simulink model "EPA_Jumpe_v1"  (R2018a)
settings: Solver=FixedStepDiscrete  StartTime=0.0  StopTime=inf  FixedStep=0.001  RelTol=1e-3  EnableMultiTasking=on
model workspace (MAT data in the model file):
  MCOS : class17 (value not decoded)
values from neighbouring files (symbols this model uses):
  bits_current = 12    [Init_EPA_Jumper.m]
  bits_GRF = 12    [Init_EPA_Jumper.m]
  bits_Kd = 12    [Init_EPA_Jumper.m]
  bits_Kp = 12    [Init_EPA_Jumper.m]
  bits_position = 16    [Init_EPA_Jumper.m]
  bits_velocity = 12    [Init_EPA_Jumper.m]
  deadzone_in_TIB = 0.45    [Init_EPA_Jumper.m]
  deadzone_out_TIB = 0.48    [Init_EPA_Jumper.m]
  GRF_MAX = 3.3    [Init_EPA_Jumper.m]
  GRF_MIN = 0    [Init_EPA_Jumper.m]
  k_p_TIB = 1    [Init_EPA_Jumper.m]
  KD_MAX = 5.0    (= 5)    [Init_EPA_Jumper.m]
  KD_MIN = 0.0    (= 0)    [Init_EPA_Jumper.m]
  KP_MAX = 500.0    (= 500)    [Init_EPA_Jumper.m]
  KP_MIN = 0.0    (= 0)    [Init_EPA_Jumper.m]
  P_MAX = 95.5    [Init_EPA_Jumper.m]
  P_MIN = -95.5    [Init_EPA_Jumper.m]
  PressureFilter_CutOffFreq = 50    [Init_EPA_Jumper.m]
  PressureFilter_Gain = 1    [Init_EPA_Jumper.m]
  ReadingVoltage = 5    [Init_EPA_Jumper.m]
  T_MAX = 18.0    (= 18)    [Init_EPA_Jumper.m]
  T_MIN = -18.0    (= -18)    [Init_EPA_Jumper.m]
  V_MAX = 45.0    (= 45)    [Init_EPA_Jumper.m]
  V_MIN = -45.0    (= -45)    [Init_EPA_Jumper.m]
  voltageBias_GAS = -2.3721    [Init_EPA_Jumper.m]
  voltageBias_GL = -2.2892    [Init_EPA_Jumper.m]
  voltageBias_HAM = -2.3721    [Init_EPA_Jumper.m]
  voltageBias_IL = -2.3721    [Init_EPA_Jumper.m]
  voltageBias_POP = -2.3721    [Init_EPA_Jumper.m]
  voltageBias_RF = -2.3721    [Init_EPA_Jumper.m]
  voltageBias_SOL = -2.3721    [Init_EPA_Jumper.m]
  voltageBias_TIB = -2.3721    [Init_EPA_Jumper.m]
  voltageBias_VAS = -2.3721    [Init_EPA_Jumper.m]
  voltageMultiplier_GAS = 2.4915    [Init_EPA_Jumper.m]
  voltageMultiplier_GL = 2.5259    [Init_EPA_Jumper.m]
  voltageMultiplier_HAM = 2.4915    [Init_EPA_Jumper.m]
  voltageMultiplier_IL = 2.4915    [Init_EPA_Jumper.m]
  voltageMultiplier_POP = 2.4915    [Init_EPA_Jumper.m]
  voltageMultiplier_RF = 2.4915    [Init_EPA_Jumper.m]
  voltageMultiplier_SOL = 2.4915    [Init_EPA_Jumper.m]
  voltageMultiplier_TIB = 2.4915    [Init_EPA_Jumper.m]
  voltageMultiplier_VAS = 2.4915    [Init_EPA_Jumper.m]
  VoltageResolution = 1024.0    (= 1024)    [Init_EPA_Jumper.m]
libraries: xpcethercatlib x75, simulink x10, peGeneralControl x9, slrtlib x9
(part 3 of 3)

== matlab function EPA_Jumpe_v1/Safety /MATLAB Function ==
  data: Hip_motor_safe output; Knee_motor_safe output; Motors_safe output; flag output; Hip_Position input; Knee_Position input; flag_1 input
function [Hip_motor_safe, Knee_motor_safe,Motors_safe,flag]= fcn(Hip_Position, Knee_Position, flag_1)

flag = flag_1;
if flag == 0
    if Hip_Position >= -50 && Hip_Position <50
        Hip_motor_safe = 1;
    else
        Hip_motor_safe = 0;   
        flag = 1;
    end
    if Knee_Position >= -10 && Knee_Position <110
        Knee_motor_safe = 1;
    else
        Knee_motor_safe = 0;  
        flag = 1;
    end
    Motors_safe = double(Hip_motor_safe & Knee_motor_safe);
else
    if Hip_Position >= -50 && Hip_Position <50
        Hip_motor_safe = 1;
    else
        Hip_motor_safe = 0;   
        flag = 1;
    end

    if Knee_Position >= -5 && Knee_Position <110
        Knee_motor_safe = 1;
    else
        Knee_motor_safe = 0;  
        flag = 1;
    end
    Motors_safe = 0;
end

end

== matlab function EPA_Jumpe_v1/High Level Control/MATLAB Function ==
  data: isFligth input; Hip_mode output; Knee_mode output
function [Hip_mode, Knee_mode] = fcn(isFligth)

if isFligth == 1
    Hip_mode = 1;
    Knee_mode = 1;
elseif isFligth == 0
    Hip_mode = 2;
    Knee_mode = 2;
else
    Hip_mode = 0;
    Knee_mode = 0;
end
end

== matlab function EPA_Jumpe_v1/Ethernet Communication/Inputs/PAMs Slave/MATLAB Function ==
  data: sensorValue input; pressure output; voltageMultiplier_TIB parameter; voltageBias_TIB parameter; ReadingVoltage parameter; VoltageResolution parameter
function pressure   = fcn(sensorValue,voltageMultiplier_TIB, voltageBias_TIB,ReadingVoltage, VoltageResolution)
pressure   = PressureSensor(sensorValue,voltageMultiplier_TIB, voltageBias_TIB,ReadingVoltage,VoltageResolution);
end

== matlab function EPA_Jumpe_v1/Ethernet Communication/Inputs/PAMs Slave/MATLAB Function1 ==
  data: sensorValue input; pressure output; voltageMultiplier_SOL parameter; voltageBias_SOL parameter; ReadingVoltage parameter; VoltageResolution parameter
function pressure   = fcn(sensorValue,voltageMultiplier_SOL, voltageBias_SOL,ReadingVoltage, VoltageResolution)
pressure   = PressureSensor(sensorValue,voltageMultiplier_SOL, voltageBias_SOL,ReadingVoltage,VoltageResolution);
end

== matlab function EPA_Jumpe_v1/Ethernet Communication/Inputs/PAMs Slave/MATLAB Function2 ==
  data: sensorValue input; pressure output; voltageMultiplier_GAS parameter; voltageBias_GAS parameter; ReadingVoltage parameter; VoltageResolution parameter
function pressure   = fcn(sensorValue,voltageMultiplier_GAS, voltageBias_GAS,ReadingVoltage, VoltageResolution)
pressure   = PressureSensor(sensorValue,voltageMultiplier_GAS, voltageBias_GAS,ReadingVoltage,VoltageResolution);
end

== matlab function EPA_Jumpe_v1/Ethernet Communication/Inputs/PAMs Slave/MATLAB Function3 ==
  data: sensorValue input; pressure output; voltageMultiplier_VAS parameter; voltageBias_VAS parameter; ReadingVoltage parameter; VoltageResolution parameter
function pressure   = fcn(sensorValue,voltageMultiplier_VAS, voltageBias_VAS,ReadingVoltage, VoltageResolution)
pressure   = PressureSensor(sensorValue,voltageMultiplier_VAS, voltageBias_VAS,ReadingVoltage,VoltageResolution);
end

== matlab function EPA_Jumpe_v1/Ethernet Communication/Inputs/PAMs Slave/MATLAB Function4 ==
  data: sensorValue input; pressure output; voltageMultiplier_POP parameter; voltageBias_POP parameter; ReadingVoltage parameter; VoltageResolution parameter
function pressure   = fcn(sensorValue,voltageMultiplier_POP, voltageBias_POP,ReadingVoltage, VoltageResolution)
pressure   = PressureSensor(sensorValue,voltageMultiplier_POP, voltageBias_POP,ReadingVoltage,VoltageResolution);
end

== matlab function EPA_Jumpe_v1/Ethernet Communication/Inputs/PAMs Slave/MATLAB Function5 ==
  data: sensorValue input; pressure output; voltageMultiplier_RF parameter; voltageBias_RF parameter; ReadingVoltage parameter; VoltageResolution parameter
function pressure   = fcn(sensorValue,voltageMultiplier_RF, voltageBias_RF,ReadingVoltage, VoltageResolution)
pressure   = PressureSensor(sensorValue,voltageMultiplier_RF, voltageBias_RF,ReadingVoltage,VoltageResolution);
end

== matlab function EPA_Jumpe_v1/Ethernet Communication/Inputs/PAMs Slave/MATLAB Function6 ==
  data: sensorValue input; pressure output; voltageMultiplier_HAM parameter; voltageBias_HAM parameter; ReadingVoltage parameter; VoltageResolution parameter
function pressure   = fcn(sensorValue,voltageMultiplier_HAM, voltageBias_HAM,ReadingVoltage, VoltageResolution)
pressure   = PressureSensor(sensorValue,voltageMultiplier_HAM, voltageBias_HAM,ReadingVoltage,VoltageResolution);
end

== matlab function EPA_Jumpe_v1/Ethernet Communication/Inputs/PAMs Slave/MATLAB Function7 ==
  data: sensorValue input; pressure output; voltageMultiplier_IL parameter; voltageBias_IL parameter; ReadingVoltage parameter; VoltageResolution parameter
function pressure   = fcn(sensorValue,voltageMultiplier_IL, voltageBias_IL,ReadingVoltage, VoltageResolution)
pressure   = PressureSensor(sensorValue,voltageMultiplier_IL, voltageBias_IL,ReadingVoltage,VoltageResolution);
end

== matlab function EPA_Jumpe_v1/Ethernet Communication/Inputs/PAMs Slave/MATLAB Function8 ==
  data: sensorValue input; pressure output; voltageMultiplier_GL parameter; voltageBias_GL parameter; ReadingVoltage parameter; VoltageResolution parameter
function pressure   = fcn(sensorValue,voltageMultiplier_GL, voltageBias_GL,ReadingVoltage, VoltageResolution)
pressure   = PressureSensor(sensorValue,voltageMultiplier_GL, voltageBias_GL,ReadingVoltage,VoltageResolution);
end

== matlab function EPA_Jumpe_v1/PAMs/TIB/Solenoids ==
  data: control input; intake output; inside_deadzone input; outtake output; inside_deadzone_1 output; PAMs_on input; System_on input; deadzone_in_TIB parameter; deadzone_out_TIB parameter; depressurize input
function [intake, outtake,inside_deadzone_1] = fcn(control, inside_deadzone, PAMs_on,System_on, deadzone_in_TIB, deadzone_out_TIB, depressurize)

[intake, outtake,inside_deadzone_1] = Solenoid(control, inside_deadzone, deadzone_in_TIB, deadzone_out_TIB,PAMs_on,System_on,depressurize);
    
  
end

== matlab function EPA_Jumpe_v1/PAMs/SOL/Solenoids ==
  data: control input; intake output; inside_deadzone input; outtake output; inside_deadzone_1 output; deadzone_in input; deadzone_out input; PAMs_on input; System_on input; depressurize input
function [intake, outtake,inside_deadzone_1] = fcn(control, inside_deadzone, deadzone_in, deadzone_out,PAMs_on,System_on,depressurize)

[intake, outtake,inside_deadzone_1] = Solenoid(control, inside_deadzone, deadzone_in, deadzone_out,PAMs_on,System_on,depressurize);
    
  
end

== matlab function EPA_Jumpe_v1/PAMs/GAS/Solenoids ==
  data: control input; intake output; inside_deadzone input; outtake output; inside_deadzone_1 output; deadzone_in input; deadzone_out input; PAMs_on input; System_on input; depressurize input
function [intake, outtake,inside_deadzone_1] = fcn(control, inside_deadzone, deadzone_in, deadzone_out,PAMs_on,System_on,depressurize)

[intake, outtake,inside_deadzone_1] = Solenoid(control, inside_deadzone, deadzone_in, deadzone_out,PAMs_on,System_on,depressurize);
    
  
end

== matlab function EPA_Jumpe_v1/PAMs/VAS/Solenoids ==
  data: control input; intake output; inside_deadzone input; outtake output; inside_deadzone_1 output; deadzone_in input; deadzone_out input; PAMs_on input; System_on input; depressurize input
function [intake, outtake,inside_deadzone_1] = fcn(control, inside_deadzone, deadzone_in, deadzone_out,PAMs_on,System_on,depressurize)

[intake, outtake,inside_deadzone_1] = Solenoid(control, inside_deadzone, deadzone_in, deadzone_out,PAMs_on,System_on,depressurize);
    
  
end

== matlab function EPA_Jumpe_v1/PAMs/POP/Solenoids ==
  data: control input; intake output; inside_deadzone input; outtake output; inside_deadzone_1 output; deadzone_in input; deadzone_out input; PAMs_on input; System_on input; depressurize input
function [intake, outtake,inside_deadzone_1] = fcn(control, inside_deadzone, deadzone_in, deadzone_out,PAMs_on,System_on,depressurize)

[intake, outtake,inside_deadzone_1] = Solenoid(control, inside_deadzone, deadzone_in, deadzone_out,PAMs_on,System_on,depressurize);
    
  
end

== matlab function EPA_Jumpe_v1/PAMs/RF/Solenoids ==
  data: control input; intake output; inside_deadzone input; outtake output; inside_deadzone_1 output; deadzone_in input; deadzone_out input; PAMs_on input; System_on input; depressurize input
function [intake, outtake,inside_deadzone_1] = fcn(control, inside_deadzone, deadzone_in, deadzone_out,PAMs_on,System_on,depressurize)

[intake, outtake,inside_deadzone_1] = Solenoid(control, inside_deadzone, deadzone_in, deadzone_out,PAMs_on,System_on,depressurize);
    
  
end

== matlab function EPA_Jumpe_v1/PAMs/HAM/Solenoids ==
  data: control input; intake output; inside_deadzone input; outtake output; inside_deadzone_1 output; deadzone_in input; deadzone_out input; PAMs_on input; System_on input; depressurize input
function [intake, outtake,inside_deadzone_1] = fcn(control, inside_deadzone, deadzone_in, deadzone_out,PAMs_on,System_on,depressurize)

[intake, outtake,inside_deadzone_1] = Solenoid(control, inside_deadzone, deadzone_in, deadzone_out,PAMs_on,System_on,depressurize);
    
  
end

== matlab function EPA_Jumpe_v1/PAMs/IL/Solenoids ==
  data: control input; intake output; inside_deadzone input; outtake output; inside_deadzone_1 output; deadzone_in input; deadzone_out input; PAMs_on input; System_on input; depressurize input
function [intake, outtake,inside_deadzone_1] = fcn(control, inside_deadzone, deadzone_in, deadzone_out,PAMs_on,System_on,depressurize)

[intake, outtake,inside_deadzone_1] = Solenoid(control, inside_deadzone, deadzone_in, deadzone_out,PAMs_on,System_on,depressurize);
    
  
end

== matlab function EPA_Jumpe_v1/PAMs/GL/Solenoids ==
  data: control input; intake output; inside_deadzone input; outtake output; inside_deadzone_1 output; deadzone_in input; deadzone_out input; PAMs_on input; System_on input; depressurize input
function [intake, outtake,inside_deadzone_1] = fcn(control, inside_deadzone, deadzone_in, deadzone_out,PAMs_on,System_on,depressurize)

[intake, outtake,inside_deadzone_1] = Solenoid(control, inside_deadzone, deadzone_in, deadzone_out,PAMs_on,System_on,depressurize);
    
  
end

== matlab function EPA_Jumpe_v1/Ethernet Communication/Inputs/GRF Slave/GRFz /Hip Position Transformation ==
  data: x_int input; GRF_z output; GRF_MIN parameter; GRF_MAX parameter; bits_GRF parameter
function GRF_z = uint_to_float(x_int, GRF_MIN, GRF_MAX, bits_GRF)
    GRF_z = uint_to_float(x_int, GRF_MIN, GRF_MAX, bits_GRF);
end

== matlab function EPA_Jumpe_v1/Ethernet Communication/Inputs/GRF Slave/GRFy /Hip Position Transformation ==
  data: x_int input; GRF_y output; GRF_MIN parameter; GRF_MAX parameter; bits_GRF parameter
function GRF_y = uint_to_float(x_int, GRF_MIN, GRF_MAX, bits_GRF)
    GRF_y = uint_to_float(x_int, GRF_MIN, GRF_MAX, bits_GRF);
end

== matlab function EPA_Jumpe_v1/Ethernet Communication/Inputs/GRF Slave/GRFx /Hip Position Transformation ==
  data: x_int input; GRF_x output; GRF_MIN parameter; GRF_MAX parameter; bits_GRF parameter
function GRF_x = uint_to_float(x_int, GRF_MIN, GRF_MAX, bits_GRF)
    GRF_x = uint_to_float(x_int, GRF_MIN, GRF_MAX, bits_GRF);
end
